simulink model "task_2_schem"  (R2024a)
settings: Solver=VariableStepAuto  StartTime=0.0  StopTime=100  RelTol=1e-3
undefined symbols (not defined in the file): B_g, C_y, init_g1, over_F, T
settings Model: Creator=user  LastModifiedBy=user

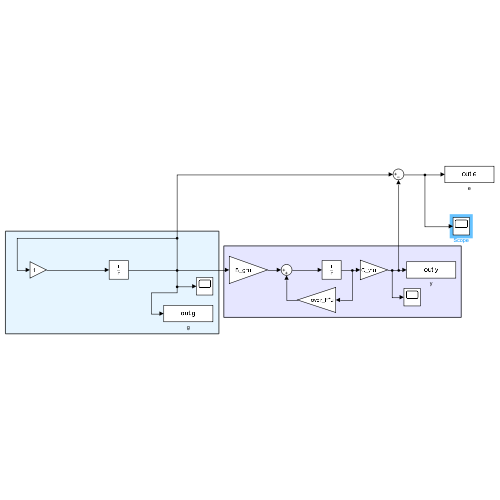
[thumbnail: Simulink's stored preview of the top-level diagram]
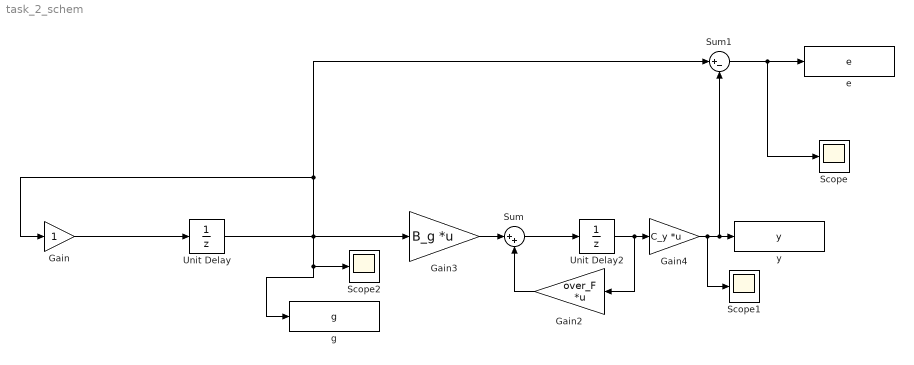
== system task_2_schem ==
  Gain : Gain
  Gain2 : Gain  Gain=over_F  Multiplication=Matrix(K*u)
  Gain3 : Gain  Gain=B_g  Multiplication=Matrix(K*u)
  Gain4 : Gain  Gain=C_y  Multiplication=Matrix(K*u)
  Scope : Scope
  Scope1 : Scope
  Scope2 : Scope
  Sum : Sum  Inputs=|++
  Sum1 : Sum  Inputs=|+-
  Unit Delay : UnitDelay  InitialCondition=init_g1  SampleTime=T  HasFrameUpgradeWarning=on
  Unit Delay2 : UnitDelay  InitialCondition=[0;0;2.8]  SampleTime=T  HasFrameUpgradeWarning=on
  e : ToWorkspace  VariableName=e  SaveFormat=Timeseries  SampleTime=-1
  g : ToWorkspace  VariableName=g  SaveFormat=Timeseries  SampleTime=-1
  y : ToWorkspace  VariableName=y  SaveFormat=Timeseries  SampleTime=-1
  wires:
  Gain/1 -> Unit Delay/1
  Unit Delay/1 -> Gain3/1, Sum1/1, Gain/1, Scope2/1, g/1
  Gain3/1 -> Sum/1
  Gain2/1 -> Sum/2
  Sum/1 -> Unit Delay2/1
  Unit Delay2/1 -> Gain4/1, Gain2/1
  Gain4/1 -> Scope1/1, Sum1/2, y/1
  Sum1/1 -> e/1, Scope/1
